simulink model "InputProcessing"  (R2018a)
settings: configuration reference "ConfigSet" (kept outside this file)
libraries: CustomLibrary x1, simulink x1
settings Model: DataDictionary=CANLights.sldd  ExtModeTrigDuration=2  Creator=The MathWorks, Inc.  LastModifiedBy=jonathancoulter

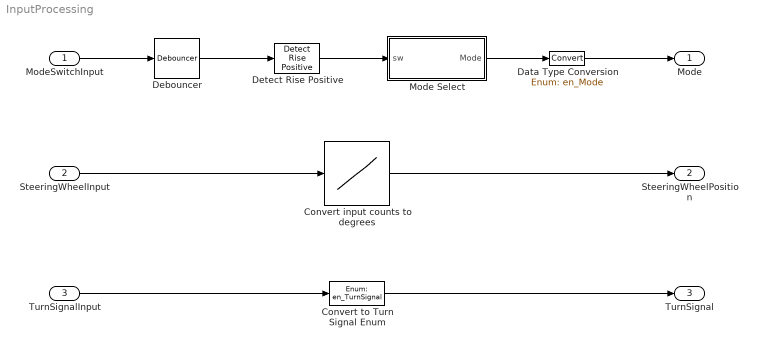
== system InputProcessing ==
  ModeSwitchInput : Inport  OutDataTypeStr=boolean
  SteeringWheelInput : Inport  Port=2  OutDataTypeStr=uint16
  TurnSignalInput : Inport  Port=3  OutDataTypeStr=uint16
  Convert input counts to degrees : Lookup_n-D  NumberOfTableDimensions=1  DataSpecification=Lookup table object  LookupTableObject=SteeringWheelAngle_LUT  BreakpointsForDimension1=[0 1023]  Table=[-90 90]  ExtrapMethod=Clip  UseLastTableValue=on  InternalRulePriority=Speed  OutDataTypeStr=int16  RndMeth=Simplest  InputSameDT=on
  Convert to Turn Signal Enum : DataTypeConversion  OutDataTypeStr=Enum: en_TurnSignal
  Data Type Conversion : DataTypeConversion  OutDataTypeStr=Enum: en_Mode
  Debouncer : CustomLibrary/Debouncer
      settings: SourceProductName=Custom Blocks
  Detect Rise Positive : simulink/Logic and Bit Operations/Detect Rise Positive  vinit=false  OutDataTypeStr=boolean
  Mode Select : Stateflow chart  TreatAsAtomicUnit=on
  Mode : Outport
  SteeringWheelPosition : Outport  Port=2
  TurnSignal : Outport  Port=3
  wires:
  TurnSignalInput/1 -> Convert to Turn Signal Enum/1
  SteeringWheelInput/1 -> Convert input counts to degrees/1
  Convert input counts to degrees/1 -> SteeringWheelPosition/1
  Convert to Turn Signal Enum/1 -> TurnSignal/1
  ModeSwitchInput/1 -> Debouncer/1
  Mode Select/1(Mode) -> Data Type Conversion/1
  Debouncer/1 -> Detect Rise Positive/1
  Detect Rise Positive/1 -> Mode Select/1(sw)
  Data Type Conversion/1 -> Mode/1

== stateflow chart InputProcessing/Mode Select ==
  state Off
    en:
    Mode = 0;
  state Next_Mode
    en:
    Mode = Mode + 1;
  (default) -> Off
  Off -> Next_Mode : [sw == true]
  Next_Mode -> Off [order 2] : [sw == true]
  Next_Mode -> Next_Mode [order 1] : before(750, msec)
      | [sw == true && Mode < en_Mode.On]
  data: sw input boolean; Mode output uint8 size=1; NoOfModes parameter
